simulink model "FULL_Variable_Frequency_Driven_Asynchronous_Motor"  (R2024b)
settings: Solver=VariableStepAuto  StartTime=0.0  StopTime=10.0  RelTol=1e-3
undefined symbols (not defined in the file): DiscIntNeverNeededParam
libraries: spsDiodeLib x6, spsSeriesRLCBranchLib x3, spsAsynchronousMachineSIUnitsLib x1, spsPWMGenerator2LevelLib x1, spsThreePhaseVIMeasurementLib x1, spsThreePhaseSourceLib x1, spsUniversalBridgeLib x1, spspowerguiLib x1
settings Model: Creator=kosta  LastModifiedBy=kosta

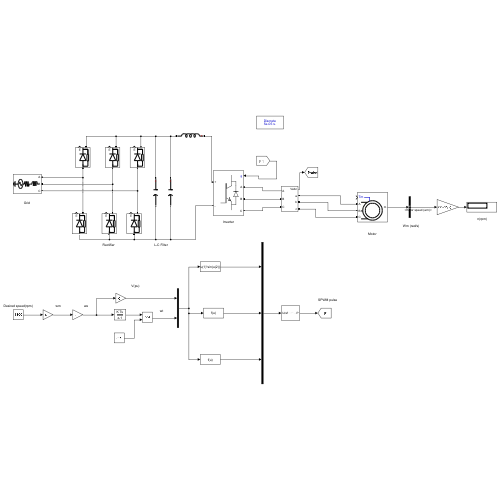
[thumbnail: Simulink's stored preview of the top-level diagram]
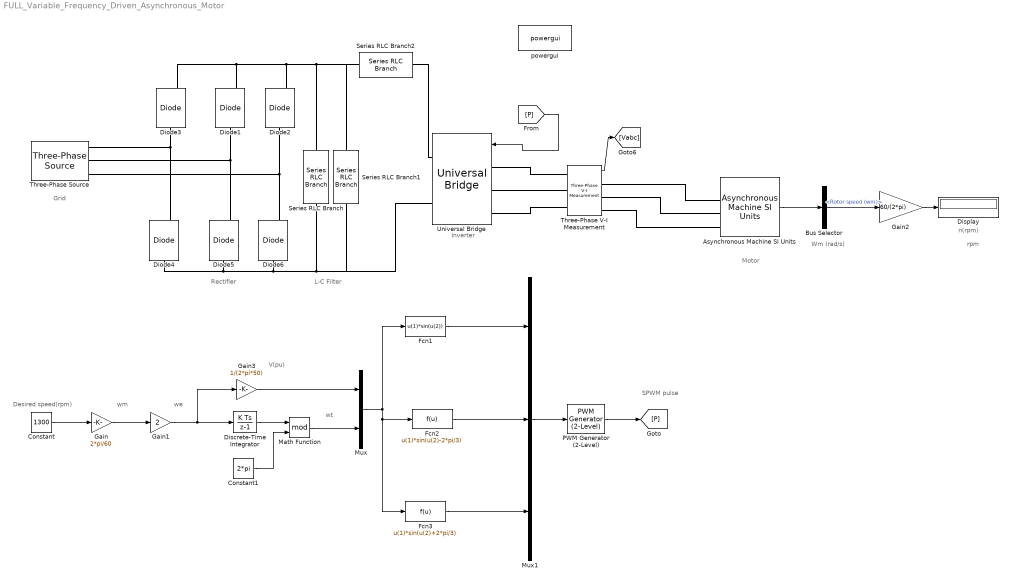
== system FULL_Variable_Frequency_Driven_Asynchronous_Motor ==
  note: Grid
  note: Motor
  note: rpm
  note: Wm (rad/s)
  note: n(rpm)
  note: Desired speed(rpm)
  note: wm
  note: we
  note: V(pu)
  note: wt
  note: SPWM pulse
  note: Rectifier
  note: L-C Filter
  note: Inverter
  Asynchronous Machine SI Units : spsAsynchronousMachineSIUnitsLib/Asynchronous Machine SI Units  RotorType=Squirrel-cage  PresetModel="15:  5.4 HP (4KW)   400 V  50Hz 1430 RPM"  MechanicalLoad=Torque Tm  ShowDetailedParameters=on  ReferenceFrame=Rotor  Units=SI  MeasurementBus=off  NominalParameters=[4000 400 50]  VoltageRatio=1  Stator=[1.405 0.005839]  Rotor=[1.395 0.005839]  Cage1=[0.4155 0.002066]  Cage2=[0.4168 0.0003495]  Lm=0.1722  Mechanical=[0.0131 0.002985 2]  PolePairs=2  InitialConditions=[0 0 0 0 0 0 0 0]  SimulateSaturation=off  Saturation=[14.03593122, 27.81365428, 53.79336849, 72.68890987, 97.98006896, 148.6815601, 215.7428561, 302.9841135, 428.7778367 ; 230, 322, 414, 460, 506, 552, 598, 644, 690]  LoadFlowParameters=1492000  TsPowergui=0  TsBlock=-1  IterativeModel=Trapezoidal non iterative  IterativeDiscreteModel=Trapezoidal non iterative  Pmec=1.492e+006
  Bus Selector : BusSelector  OutputSignals=Mechanical.Rotor speed (wm)
  Constant : Constant  Value=1300
  Constant1 : Constant  Value=2*pi
  Diode{1..6} (6 alike) : spsDiodeLib/Diode  Ron=0.001  Lon=0  Vf=0.8  IC=0  UseSnubber=0  Rs=500  Cs=250e-9  Measurements=on
  Discrete-Time Integrator : DiscreteIntegrator  SampleTime=-1  ICPrevOutput=DiscIntNeverNeededParam  ICPrevScaledInput=DiscIntNeverNeededParam
  Display : Display
  Fcn1 : Fcn  Expr=u(1)*sin(u(2))
  Fcn2 : Fcn  Expr=u(1)*sin(u(2)-2*pi/3)
  Fcn3 : Fcn  Expr=u(1)*sin(u(2)+2*pi/3)
  Gain : Gain  Gain=2*pi/60
  Gain1 : Gain  Gain=2
  Gain2 : Gain  Gain=60/(2*pi)
  Gain3 : Gain  Gain=1/(2*pi*50)
  Math Function : Math  Operator=mod
  Mux : Mux  Inputs=2
  Mux1 : Mux  Inputs=3
  PWM Generator (2-Level) : spsPWMGenerator2LevelLib/PWM Generator (2-Level)  ModulatorType=Three-phase bridge (6 pulses)  ModulatorMode=Unsynchronized  Fc=20*50  Pc=90  nF=27  MinMax="[ -1  1 ]"  SamplingTechnique=Natural  ModulatingSignals=off  m=0.8  Freq=60  Phase=0  Ts=0  ShowCarrierOutport=off
  Series RLC Branch : spsSeriesRLCBranchLib/Series RLC Branch  LConnTagsString=__new0  RConnTagsString=__new0  BranchType=C  Resistance=1  Inductance=1e-3  SetiL0=off  InitialCurrent=0  Capacitance=20e-3  Setx0=off  InitialVoltage=0  Measurements=None
  Series RLC Branch1 : spsSeriesRLCBranchLib/Series RLC Branch  LConnTagsString=__new0  RConnTagsString=__new0  BranchType=C  Resistance=1  Inductance=1e-3  SetiL0=off  InitialCurrent=0  Capacitance=20e-3  Setx0=off  InitialVoltage=0  Measurements=None
  Series RLC Branch2 : spsSeriesRLCBranchLib/Series RLC Branch  LConnTagsString=__new0  RConnTagsString=__new0  BranchType=L  Resistance=1  Inductance=5e-3  SetiL0=off  InitialCurrent=0  Capacitance=20e-3  Setx0=off  InitialVoltage=0  Measurements=None
  Three-Phase V-I Measurement : spsThreePhaseVIMeasurementLib/Three-Phase V-I Measurement  VoltageMeasurement=phase-to-phase  SetLabelV=off  LabelV=Vabc  Vpu=off  VpuLL=off  CurrentMeasurement=no  SetLabelI=off  LabelI=Iabc  Ipu=off  Pbase=100e6  Vbase=500e3  OutputType=Complex  PhasorSimulation=off  PSBequivalent=0
  Three-Phase Source : spsThreePhaseSourceLib/Three-Phase Source  InternalConnection=Yg  VoltagePhases=off  Voltage=400  PhaseAngle=0  Voltage_phases=[25e3 25e3 25e3]/sqrt(3)  PhaseAngles_phases=[0 -120 +120]  Frequency=50  NonIdealSource=on  SpecifyImpedance=off  Resistance=0.8929  Inductance=16.58e-3  ShortCircuitLevel=100e6  BaseVoltage=25e3  XRratio=7  BusType=swing  Pref=10e3  Qref=0  Prefabc=[10e3, 10e3, 10e3]  Qrefabc=[0, 0, 0]  Qmin=-inf  Qmax=inf
  Universal Bridge : spsUniversalBridgeLib/Universal Bridge  Arms=3  SnubberResistance=1e5  SnubberCapacitance=inf  Device=IGBT / Diodes  Ron=1e-3  Lon=0  ForwardVoltages="[  0  0  ]"  ForwardVoltage=0  GTOparameters=[ 10e-6 , 20e-6 ]  IGBTparameters=[ 1e-6 , 2e-6 ]  Measurements=None  Measurements_2=None  converterType=Rectifier
  powergui : spspowerguiLib/powergui  Priority=1  SimulationMode=Discrete  SampleTime=50e-6  frequency=60  Iterations=50  frequencyindice=50  Pbase=100e6  ErrMax=1e-4  UnitsV=kV  UnitsW=MW  buscounter=0  FunctionMessages=off  echomessages=off  EnableUseOfTLC=off  CurrentSourceSwitches=off  DisableSnubberDevices=off  DisableRonSwitches=off  DisableVfSwitches=off  DisplayEquations=off  AutomaticDiscreteSolvers=off  SolverType=Tustin/Backward Euler (TBE)  Interpol=off  ExternalGateDelay=off  methode=off  Ts=100  x0status=blocks  SPID=on  SwTol=0  HookPort=off  NonlinearTolerance=1e-4  nMaxIteration=100  ContinueOnMaxIteration=off  RestoreLinks=warning  ResistiveCurrentMeasurement=off  Frange=[0:2:500]  Ylog=off  Xlog=on  ShowGrid=off  save=off  variable=ZData  structure=0  ZoomFFT=off  StartTime=0.0  cycles=1  DisplayStyle=1  fundamental=60  FreqAxis=off  MaxFrequency=1000  frequencyindicesteady=1  RmsSteady=1  display=off
  wires:
  Fcn2/1 -> Mux1/2
  Three-Phase V-I Measurement/1 -> [Vabc]
  Gain1/1 -> Discrete-Time Integrator/1, Gain3/1
  Discrete-Time Integrator/1 -> Math Function/1
  [P] -> Universal Bridge/1
  Bus Selector/1 -> Gain2/1  "<Rotor speed (wm)>"
  PWM Generator (2-Level)/1 -> [P]
  Gain2/1 -> Display/1
  Fcn1/1 -> Mux1/1
  Gain/1 -> Gain1/1
  Gain3/1 -> Mux/1
  Asynchronous Machine SI Units/1 -> Bus Selector/1
  Mux/1 -> Fcn3/1, Fcn2/1, Fcn1/1
  Fcn3/1 -> Mux1/3
  Constant/1 -> Gain/1
  Math Function/1 -> Mux/2
  Mux1/1 -> PWM Generator (2-Level)/1
  Constant1/1 -> Math Function/2
  connections:
  Universal Bridge/LConn1 -- Three-Phase V-I Measurement/LConn1
  Asynchronous Machine SI Units/LConn3 -- Three-Phase V-I Measurement/RConn3
  Universal Bridge/LConn3 -- Three-Phase V-I Measurement/LConn3
  Universal Bridge/LConn2 -- Three-Phase V-I Measurement/LConn2
  Asynchronous Machine SI Units/LConn2 -- Three-Phase V-I Measurement/RConn2
  Three-Phase V-I Measurement/RConn1 -- Asynchronous Machine SI Units/LConn1
  Diode3/RConn1 -- Series RLC Branch2/RConn1 -- Series RLC Branch1/LConn1 -- Series RLC Branch/LConn1 -- Diode2/RConn1 -- Diode1/RConn1
  Diode4/LConn1 -- Series RLC Branch1/RConn1 -- Universal Bridge/RConn2 -- Series RLC Branch/RConn1 -- Diode6/LConn1 -- Diode5/LConn1
  Diode3/LConn1 -- Three-Phase Source/RConn1 -- Diode4/RConn1
  Diode1/LConn1 -- Three-Phase Source/RConn2 -- Diode5/RConn1
  Diode2/LConn1 -- Three-Phase Source/RConn3 -- Diode6/RConn1
  Series RLC Branch2/LConn1 -- Universal Bridge/RConn1
